simulink model "part1"  (R2024b)
settings: Solver=VariableStepAuto  StartTime=0.0  StopTime=1500  RelTol=1e-3
values from neighbouring files (symbols this model uses):
  A_f = diag([1/t1 1/t2 1/t3])    [reference_model.m]
  Gamma = diag([w1^2, w2^2, w3^2])    [reference_model.m]
  Kd = diag([Kd_t(1,1), Kd_t(2,2), Kd_t(3,3)])    [PID.m]
  Ki = diag([Ki_t(1,1), Ki_t(2,2), Ki_t(3,3)])    [PID.m]
  Kp = diag([Kp_t(1,1), Kp_t(2,2), Kp_t(3,3)])    [PID.m]
  Omega = diag([2*zeta1*w1, 2*zeta2*w2, 2*zeta3*w3])    [reference_model.m]
  step1 = 50    [reference_model.m]
  step2 = 1.4    [reference_model.m]
  step3 = 1.2    [reference_model.m]
  W = diag([10, 1, 1, 10, 1, 1, 1, 1])    [thrust_allocation.m]
  xpos = [thrusters.xposition]    [thrust_allocation.m]
  ypos = [thrusters.yposition]    [thrust_allocation.m]
undefined symbols (not defined in the file or in its folder): alpha, C_pitch, C_roll, C_yaw, Cx, Cy, Cz, Hoerner, magnitude, thrusters, vessel
libraries: simulink x4, marine_gnc x3, marine_hydro x1
settings Model: Creator=jonbjor  LastModifiedBy=audun
settings SolverCC: AlgebraicLoopSolver=TrustRegion
settings DataIOCC: ReturnWorkspaceOutputs=off
settings DebuggingCC: UnconnectedInputMsg=warning  UnconnectedOutputMsg=warning  UnconnectedLineMsg=warning  ArithmeticOperatorsInVariantConditions=warning
settings ModelReferenceCC: EnableRefExpFcnMdlSchedulingChecks=on
settings SFSimCC: SimUseLocalCustomCode=off  CustomCodeUndefinedFunction=UseInterfaceOnly
settings RTWCC: RTWUseLocalCustomCode=off  GPUComputeCapability=3.5  DLArmComputeVersion=19.05

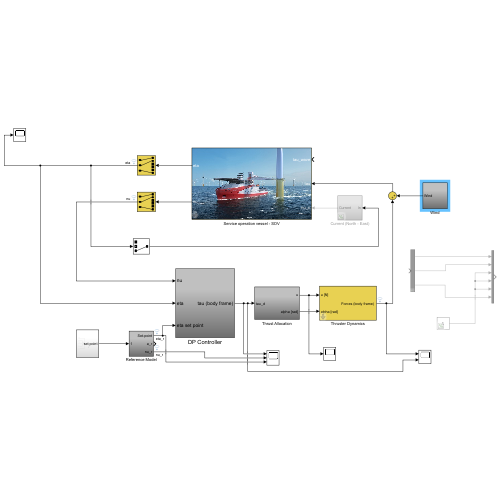
[thumbnail: Simulink's stored preview of the top-level diagram]
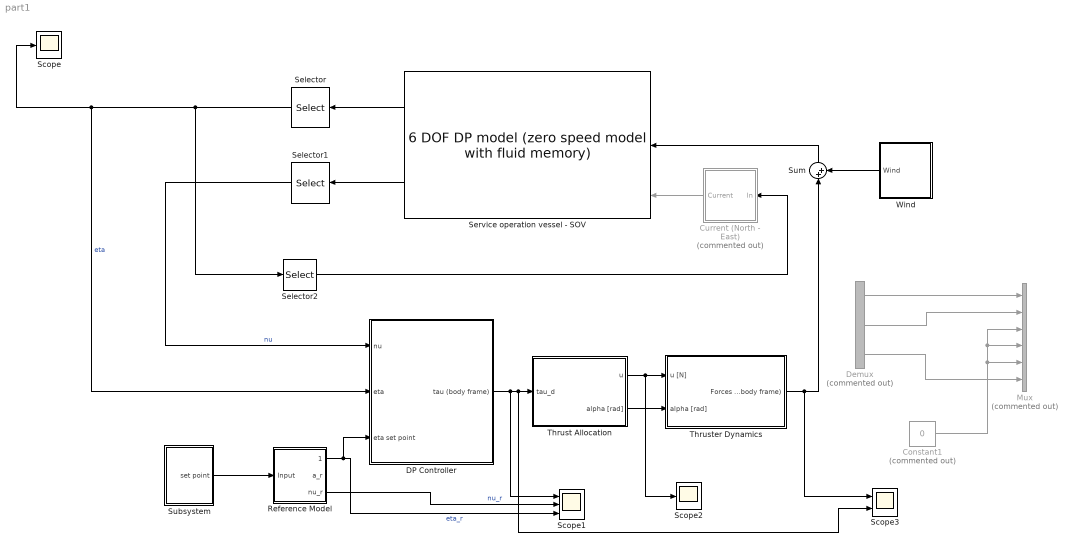
== system part1 ==
  Constant1 : Constant  Commented=on  Value=0
  Current (North - East) : Subsystem  Commented=on
  DP Controller : Subsystem
  Demux : Demux  Commented=on  Outputs=3
  Mux : Mux  Commented=on  Inputs=6
  Reference Model : Subsystem
  Scope : Scope
  Scope1 : Scope  NumInputPorts=3
  Scope2 : Scope
  Scope3 : Scope  NumInputPorts=2
  Selector : Selector  InputPortWidth=6  IndexOptions=Index vector (dialog)  Indices=[1 2 6]  OutputSizes=1
  Selector1 : Selector  InputPortWidth=6  IndexOptions=Index vector (dialog)  Indices=[1 2 6]  OutputSizes=1
  Selector2 : Selector  InputPortWidth=3  IndexOptions=Index vector (dialog)  Indices=[3]  OutputSizes=1
  Service operation vessel - SOV : marine_hydro/Hydro Library/6 DOF DP model  (zero speed model with fluid memory)  ABC=vesselABC  rho=1025  Axc=0.9*vessel.main.T*vessel.main.B  Ayc=0.9*vessel.main.T*vessel.main.Lpp  CX=1  CY_2D=Hoerner(vessel.main.B,vessel.main.T)  Bv=vessel.Bv  mask(6 DOF zero speed model){}
      link override "Integrator1 ": InitialCondition=nu0
      link override Integrator2: InitialCondition=eta0
      settings: SourceProductName=MSS Hydro
      mask Display:
      | image('SOV.jpg');
      | color('white'); port_label('output', 1, 'eta')
      | color('white'); port_label('output', 2, 'nu')
      | color('white'); port_label('input', 1, 'tau_wave')
      | color('white'); port_label('input', 2, 'tau')
      | color('white'); port_label('input', 3, 'nu_c')
  Subsystem : Subsystem
  Sum : Sum  Inputs=|++
  Thrust Allocation : Subsystem
  Thruster Dynamics : Subsystem  mask{thrusterfault=off}
      mask prompts: thrusterfault "Fault on thruster #2 and #4?"
  Wind : Subsystem
  wires:
  Thruster Dynamics/1("Forces (body frame) ") -> Scope3/1, Sum/1
  Service operation vessel - SOV/1 -> Selector/1
  Service operation vessel - SOV/2 -> Selector1/1
  Selector/1 -> Selector2/1, DP Controller/2(eta), Scope/1  "eta"
  Selector1/1 -> DP Controller/1(nu)  "nu"
  DP Controller/1(tau (body frame)) -> Scope1/1, Scope3/2, Thrust Allocation/1(tau_d)
  Wind/1(Wind) -> Sum/2
  Demux/1 -> Mux/1
  Demux/2 -> Mux/2
  Constant1/1 -> Mux/5, Mux/4, Mux/3
  Demux/3 -> Mux/6
  Thrust Allocation/1(u) -> Scope2/1, Thruster Dynamics/1(u [N])
  Thrust Allocation/2(alpha [rad]) -> Thruster Dynamics/2(alpha [rad])
  Sum/1 -> Service operation vessel - SOV/2
  Subsystem/1(set point) -> Reference Model/1(Input)
  Selector2/1 -> Current (North - East)/1(In)
  Current (North - East)/1(Current) -> Service operation vessel - SOV/3
  Reference Model/1(Set-point) -> DP Controller/3(eta set point), Scope1/3  "eta_r"
  Reference Model/3(nu_r) -> Scope1/2  "nu_r"

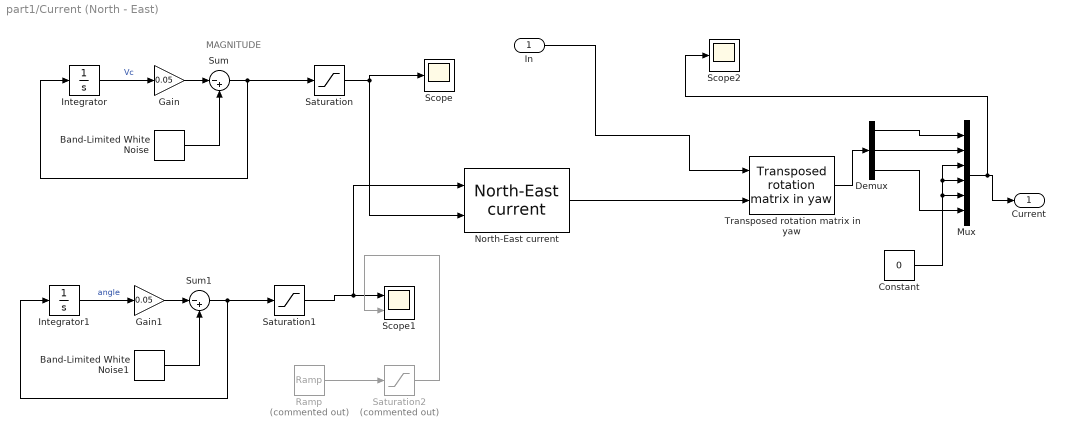
== system part1/Current (North - East) ==
  note: MAGNITUDE
  In : Inport
  Band-Limited White Noise : simulink/Sources/Band-Limited White Noise  Cov=[0.1]  Ts=0.1  seed=[23341]
  Band-Limited White Noise1 : simulink/Sources/Band-Limited White Noise  Cov=[0.1]  Ts=0.1  seed=[23341]
  Constant : Constant  Value=0
  Demux : Demux  Outputs=3
  Gain : Gain  Gain=0.05
  Gain1 : Gain  Gain=0.05
  Integrator : Integrator
  Integrator1 : Integrator
  Mux : Mux  Inputs=6
  North-East current : marine_gnc/Environment/Current/North-East current  SystemSampleTime=-1  VariantActivationTime=update diagram  AllowFlexibleInterface=on  Latency=0  AutoFrameSizeCalculation=off
      settings: SourceProductName=MSS GNC
  Ramp : simulink/Sources/Ramp  Commented=on  slope=0.3  start=0  InitialOutput=180
  Saturation : Saturate  LowerLimit=0.5
  Saturation1 : Saturate  UpperLimit=270  LowerLimit=270
  Saturation2 : Saturate  Commented=on  UpperLimit=270  LowerLimit=0
  Scope : Scope
  Scope1 : Scope  NumInputPorts=2
  Scope2 : Scope
  Sum : Sum  Inputs=|-+
  Sum1 : Sum  Inputs=|-+
  Transposed rotation matrix in yaw : marine_gnc/Models/ Kinematics/Transposed rotation  matrix in yaw
      settings: SourceProductName=MSS GNC
  Current : Outport  VectorParamsAs1DForOutWhenUnconnected=off
  wires:
  Transposed rotation matrix in yaw/1 -> Demux/1
  In/1 -> Transposed rotation matrix in yaw/1
  Demux/1 -> Mux/1
  Band-Limited White Noise1/1 -> Sum1/2
  Integrator/1 -> Gain/1  "Vc"
  Sum/1 -> Saturation/1, Integrator/1
  Gain/1 -> Sum/1
  Integrator1/1 -> Gain1/1  "angle"
  Gain1/1 -> Sum1/1
  Constant/1 -> Mux/5, Mux/4, Mux/3
  Demux/3 -> Mux/6
  Saturation/1 -> Scope/1, North-East current/2
  Saturation1/1 -> North-East current/1, Scope1/1
  Sum1/1 -> Saturation1/1, Integrator1/1
  North-East current/1 -> Transposed rotation matrix in yaw/2
  Band-Limited White Noise/1 -> Sum/2
  Mux/1 -> Scope2/1, Current/1
  Demux/2 -> Mux/2
  Ramp/1 -> Saturation2/1
  Saturation2/1 -> Scope1/2

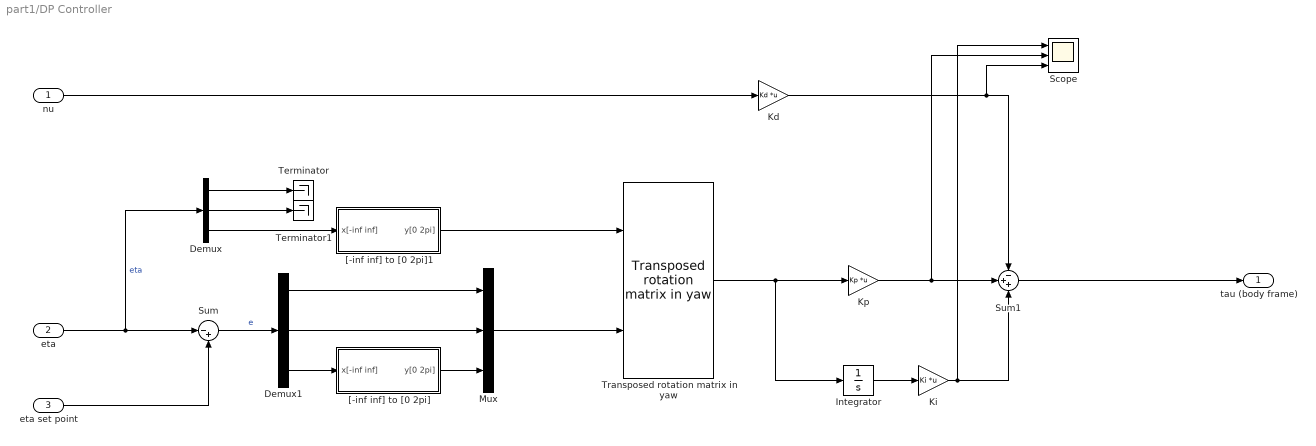
== system part1/DP Controller ==
  nu : Inport
  eta : Inport  Port=2
  eta set point : Inport  Port=3
  Demux : Demux  Outputs=3
  Demux1 : Demux  Outputs=3
  Integrator : Integrator
  Kd : Gain  Gain=Kd  Multiplication=Matrix(K*u)
  Ki : Gain  Gain=Ki  Multiplication=Matrix(K*u)
  Kp : Gain  Gain=Kp  Multiplication=Matrix(K*u)
  Mux : Mux  Inputs=3
  Scope : Scope  NumInputPorts=3
  Sum : Sum  Inputs=|-+
  Sum1 : Sum  Inputs=-++
  Terminator : Terminator
  Terminator1 : Terminator
  Transposed rotation matrix in yaw : marine_gnc/Models/ Kinematics/Transposed rotation  matrix in yaw
      settings: SourceProductName=MSS GNC
  "[-inf inf] to [0 2pi]" : Subsystem
  "[-inf inf] to [0 2pi]1" : Subsystem
  tau (body frame) : Outport  VectorParamsAs1DForOutWhenUnconnected=off
  wires:
  eta set point/1 -> Sum/2
  eta/1 -> Demux/1, Sum/1  "eta"
  Sum/1 -> Demux1/1  "e"
  Demux/1 -> Terminator/1
  Demux/2 -> Terminator1/1
  Demux/3 -> "[-inf inf] to [0 2pi]1"/1(x[-inf inf])
  Demux1/2 -> Mux/2
  Demux1/3 -> "[-inf inf] to [0 2pi]"/1(x[-inf inf])
  Demux1/1 -> Mux/1
  "[-inf inf] to [0 2pi]"/1(y[0 2pi]) -> Mux/3
  Integrator/1 -> Ki/1
  Ki/1 -> Scope/1, Sum1/3
  Kp/1 -> Scope/2, Sum1/2
  Kd/1 -> Scope/3, Sum1/1
  Sum1/1 -> tau (body frame)/1
  Mux/1 -> Transposed rotation matrix in yaw/2
  Transposed rotation matrix in yaw/1 -> Integrator/1, Kp/1
  nu/1 -> Kd/1
  "[-inf inf] to [0 2pi]1"/1(y[0 2pi]) -> Transposed rotation matrix in yaw/1

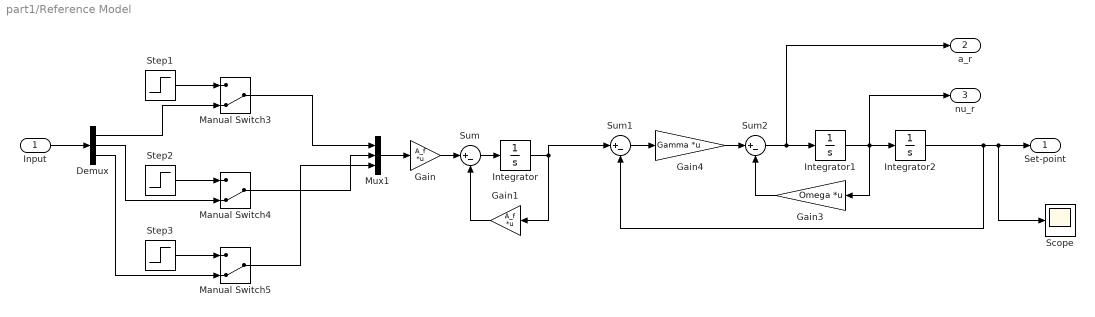
== system part1/Reference Model ==
  Input : Inport
  Demux : Demux  Outputs=3
  Gain : Gain  Gain=A_f  Multiplication=Matrix(K*u)
  Gain1 : Gain  Gain=A_f  Multiplication=Matrix(K*u)
  Gain3 : Gain  Gain=Omega  Multiplication=Matrix(K*u)
  Gain4 : Gain  Gain=Gamma  Multiplication=Matrix(K*u)
  Integrator : Integrator
  Integrator1 : Integrator
  Integrator2 : Integrator
  Manual Switch3 : ManualSwitch  CurrentSetting=0
  Manual Switch4 : ManualSwitch  CurrentSetting=0
  Manual Switch5 : ManualSwitch  CurrentSetting=0
  Mux1 : Mux  Inputs=3
  Scope : Scope
  Step1 : Step  After=step1  SampleTime=1
  Step2 : Step  After=step2  SampleTime=1
  Step3 : Step  After=step3  SampleTime=1
  Sum : Sum  Inputs=|+-
  Sum1 : Sum  Inputs=|+-
  Sum2 : Sum  Inputs=|+-
  Set-point : Outport  VectorParamsAs1DForOutWhenUnconnected=off
  a_r : Outport  Port=2
  nu_r : Outport  Port=3
  wires:
  Manual Switch3/1 -> Mux1/1
  Demux/1 -> Manual Switch3/2
  Mux1/1 -> Gain/1
  Gain4/1 -> Sum2/1
  Integrator/1 -> Sum1/1, Gain1/1
  Gain/1 -> Sum/1
  Step2/1 -> Manual Switch4/1
  Sum/1 -> Integrator/1
  Integrator2/1 -> Sum1/2, Scope/1, Set-point/1
  Gain3/1 -> Sum2/2
  Gain1/1 -> Sum/2
  Demux/3 -> Manual Switch5/2
  Manual Switch5/1 -> Mux1/3
  Demux/2 -> Manual Switch4/2
  Manual Switch4/1 -> Mux1/2
  Input/1 -> Demux/1
  Step1/1 -> Manual Switch3/1
  Step3/1 -> Manual Switch5/1
  Integrator1/1 -> Gain3/1, nu_r/1, Integrator2/1
  Sum2/1 -> a_r/1, Integrator1/1
  Sum1/1 -> Gain4/1

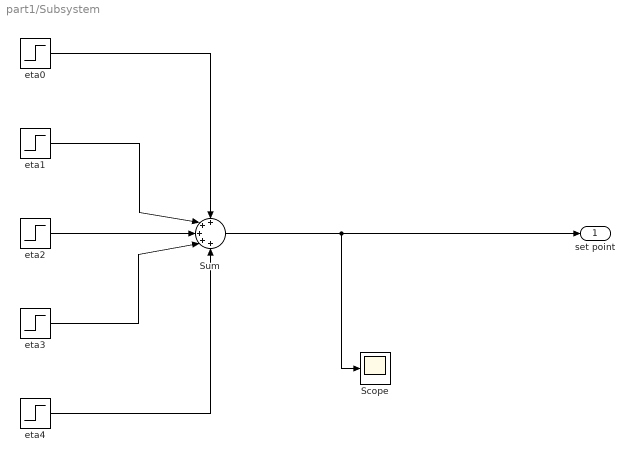
== system part1/Subsystem ==
  Scope : Scope
  Sum : Sum  Inputs=+++++
  eta0 : Step  Before=[0, 0 , 0]  After=[50, 0, 0]  SampleTime=0
  eta1 : Step  Time=301  Before=[0, 0 , 0]  After=[0, -50, 0]  SampleTime=0
  eta2 : Step  Time=601  Before=[0, 0, 0]  After=[0, 0, -pi/4]  SampleTime=0
  eta3 : Step  Time=901  Before=[0, 0, 0]  After=[-50, 0, 0]  SampleTime=0
  eta4 : Step  Time=1201  Before=[0, 0, 0]  After=[0, 50, pi/4]  SampleTime=0
  set point : Outport
  wires:
  Sum/1 -> Scope/1, set point/1
  eta0/1 -> Sum/1
  eta1/1 -> Sum/2
  eta2/1 -> Sum/3
  eta3/1 -> Sum/4
  eta4/1 -> Sum/5

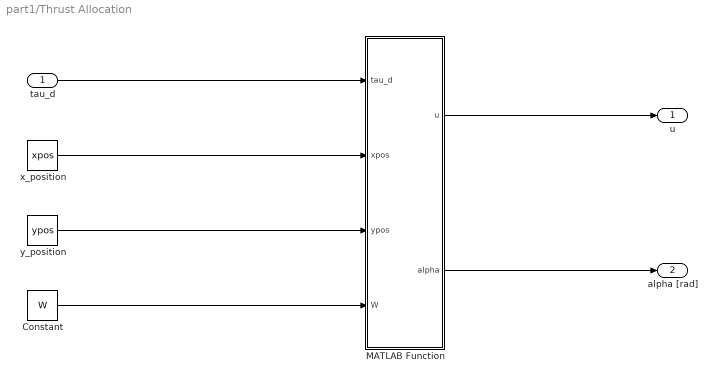
== system part1/Thrust Allocation ==
  tau_d : Inport
  Constant : Constant  Value=W
  MATLAB Function : MATLAB Function  TreatAsAtomicUnit=on
  x_position : Constant  Value=xpos
  y_position : Constant  Value=ypos
  u : Outport  VectorParamsAs1DForOutWhenUnconnected=off
  alpha [rad] : Outport  Port=2  VectorParamsAs1DForOutWhenUnconnected=off
  wires:
  tau_d/1 -> MATLAB Function/1(tau_d)
  x_position/1 -> MATLAB Function/2(xpos)
  y_position/1 -> MATLAB Function/3(ypos)
  MATLAB Function/2(alpha) -> alpha [rad]/1
  MATLAB Function/1(u) -> u/1
  Constant/1 -> MATLAB Function/4(W)

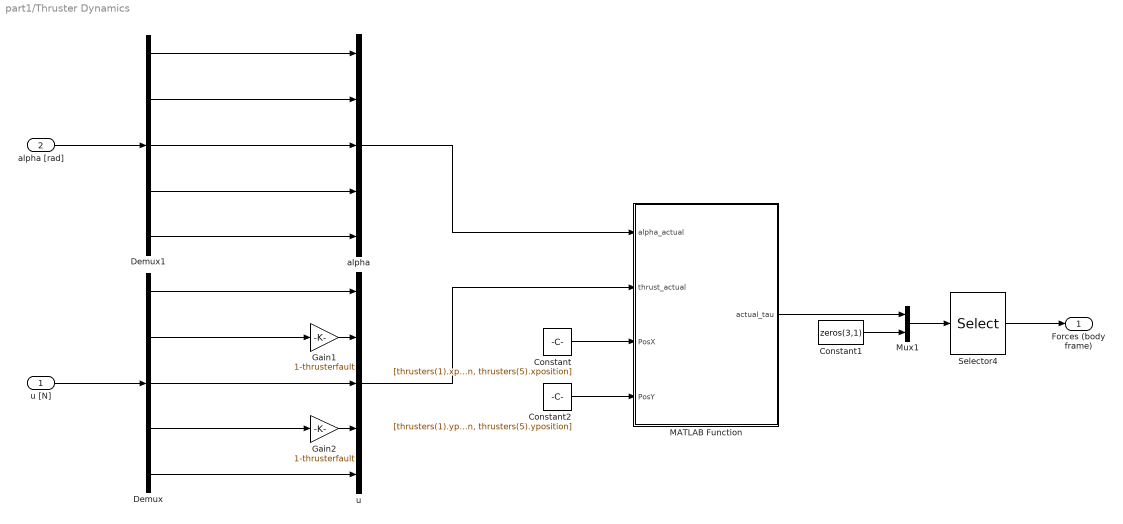
== system part1/Thruster Dynamics ==
  u [N] : Inport
  alpha [rad] : Inport  Port=2
  Constant : Constant  Value=[thrusters(1).xposition, thrusters(2).xposition, thrusters(3).xposition, thrusters(4).xposition, thrusters(5).xposition]
  Constant1 : Constant  Value=zeros(3,1)
  Constant2 : Constant  Value=[thrusters(1).yposition, thrusters(2).yposition, thrusters(3).yposition, thrusters(4).yposition, thrusters(5).yposition]
  Demux : Demux  Outputs=5
  Demux1 : Demux  Outputs=5
  Gain1 : Gain  Gain=1-thrusterfault
  Gain2 : Gain  Gain=1-thrusterfault
  MATLAB Function : MATLAB Function  TreatAsAtomicUnit=on
  Mux1 : Mux  Inputs=2
  Selector4 : Selector  InputPortWidth=6  IndexOptions=Index vector (dialog)  Indices=[1 2 4 5 6 3]  OutputSizes=1
  alpha : Mux  Inputs=5
  u : Mux  Inputs=5
  "Forces (body frame) " : Outport  VectorParamsAs1DForOutWhenUnconnected=off
  wires:
  Mux1/1 -> Selector4/1
  Constant1/1 -> Mux1/2
  Selector4/1 -> "Forces (body frame) "/1
  Gain1/1 -> u/2
  u [N]/1 -> Demux/1
  alpha [rad]/1 -> Demux1/1
  Constant/1 -> MATLAB Function/3(PosX)
  Constant2/1 -> MATLAB Function/4(PosY)
  u/1 -> MATLAB Function/2(thrust_actual)
  alpha/1 -> MATLAB Function/1(alpha_actual)
  MATLAB Function/1(actual_tau) -> Mux1/1
  Demux1/1 -> alpha/1
  Gain2/1 -> u/4
  Demux/1 -> u/1
  Demux/2 -> Gain1/1
  Demux/3 -> u/3
  Demux/4 -> Gain2/1
  Demux/5 -> u/5
  Demux1/2 -> alpha/2
  Demux1/4 -> alpha/4
  Demux1/5 -> alpha/5
  Demux1/3 -> alpha/3

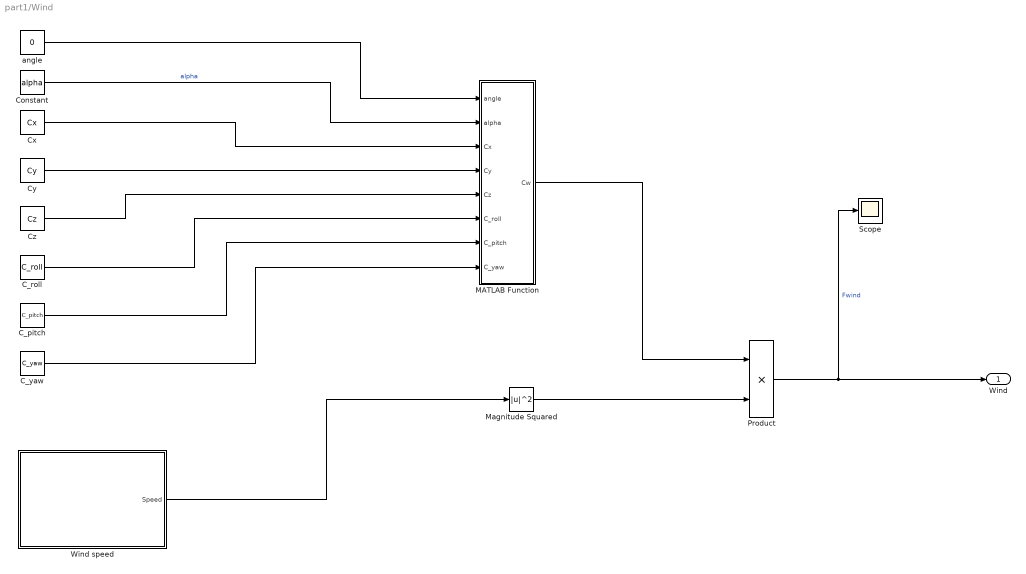
== system part1/Wind ==
  C_pitch : Constant  Value=C_pitch
  C_roll : Constant  Value=C_roll
  C_yaw : Constant  Value=C_yaw
  Constant : Constant  Value=alpha
  Cx : Constant  Value=Cx
  Cy : Constant  Value=Cy
  Cz : Constant  Value=Cz
  MATLAB Function : MATLAB Function  TreatAsAtomicUnit=on
  Magnitude Squared : Math  Operator=magnitude^2
  Product : Product
  Scope : Scope
  Wind speed : Subsystem
  angle : Constant  Value=0
  Wind : Outport  VectorParamsAs1DForOutWhenUnconnected=off
  wires:
  Cz/1 -> MATLAB Function/5(Cz)
  Cy/1 -> MATLAB Function/4(Cy)
  Cx/1 -> MATLAB Function/3(Cx)
  C_yaw/1 -> MATLAB Function/8(C_yaw)
  C_roll/1 -> MATLAB Function/6(C_roll)
  C_pitch/1 -> MATLAB Function/7(C_pitch)
  Magnitude Squared/1 -> Product/2
  Product/1 -> Wind/1, Scope/1  "Fwind"
  MATLAB Function/1(Cw) -> Product/1
  Constant/1 -> MATLAB Function/2(alpha)  "alpha"
  Wind speed/1(Speed) -> Magnitude Squared/1
  angle/1 -> MATLAB Function/1(angle)

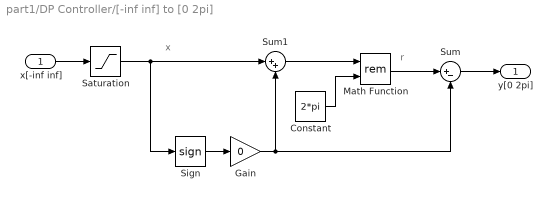
== system part1/DP Controller/[-inf inf] to [0 2pi] ==
  note: r
  note: x
  x[-inf inf] : Inport
  Constant : Constant  Value=2*pi
  Gain : Gain  Gain=0  SaturateOnIntegerOverflow=on  OutDataTypeStr=Inherit: Same as input  ParamDataTypeStr=Inherit: Same as input
  Math Function : Math  Operator=rem  SignedPower=on
  Saturation : Saturate  UpperLimit=1e10  LowerLimit=-1e10
  Sign : Signum
  Sum : Sum  Inputs=|+-  SaturateOnIntegerOverflow=on
  Sum1 : Sum  Inputs=|++  SaturateOnIntegerOverflow=on
  y[0 2pi] : Outport
  wires:
  Saturation/1 -> Sum1/1, Sign/1
  Constant/1 -> Math Function/2
  x[-inf inf]/1 -> Saturation/1
  Math Function/1 -> Sum/1
  Sum/1 -> y[0 2pi]/1
  Gain/1 -> Sum/2, Sum1/2
  Sign/1 -> Gain/1
  Sum1/1 -> Math Function/1

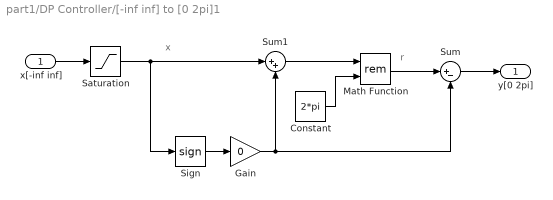
== system part1/DP Controller/[-inf inf] to [0 2pi]1 ==
  note: r
  note: x
  x[-inf inf] : Inport
  Constant : Constant  Value=2*pi
  Gain : Gain  Gain=0  SaturateOnIntegerOverflow=on  OutDataTypeStr=Inherit: Same as input  ParamDataTypeStr=Inherit: Same as input
  Math Function : Math  Operator=rem  SignedPower=on
  Saturation : Saturate  UpperLimit=1e10  LowerLimit=-1e10
  Sign : Signum
  Sum : Sum  Inputs=|+-  SaturateOnIntegerOverflow=on
  Sum1 : Sum  Inputs=|++  SaturateOnIntegerOverflow=on
  y[0 2pi] : Outport
  wires:
  Saturation/1 -> Sum1/1, Sign/1
  Constant/1 -> Math Function/2
  x[-inf inf]/1 -> Saturation/1
  Math Function/1 -> Sum/1
  Sum/1 -> y[0 2pi]/1
  Gain/1 -> Sum/2, Sum1/2
  Sign/1 -> Gain/1
  Sum1/1 -> Math Function/1

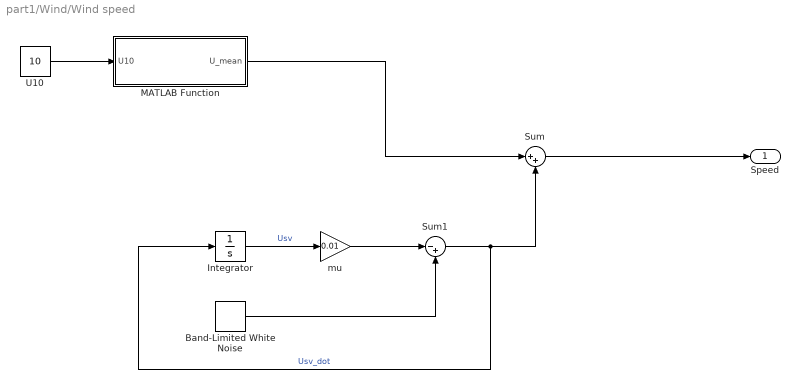
== system part1/Wind/Wind speed ==
  Band-Limited White Noise : simulink/Sources/Band-Limited White Noise  Cov=[0.1]  Ts=0.1  seed=[23341]
  Integrator : Integrator
  MATLAB Function : MATLAB Function  TreatAsAtomicUnit=on
  Sum : Sum  Inputs=|++
  Sum1 : Sum  Inputs=|-+
  U10 : Constant  Value=10
  mu : Gain  Gain=0.01
  Speed : Outport
  wires:
  U10/1 -> MATLAB Function/1(U10)
  Sum/1 -> Speed/1
  mu/1 -> Sum1/1
  Integrator/1 -> mu/1  "Usv"
  Band-Limited White Noise/1 -> Sum1/2
  Sum1/1 -> Integrator/1, Sum/2  "Usv_dot"
  MATLAB Function/1(U_mean) -> Sum/1

== matlab function part1/Thrust Allocation/MATLAB Function ==
  data: tau_d input; u output; xpos input; ypos input; alpha output; W input
function [u,alpha] = fcn(tau_d, xpos, ypos, W)

l_1 = xpos(1);
l_2x = xpos(2);
l_2y = ypos(2);
l_3 = xpos(3);
l_4x = xpos(4);
l_4y = ypos(4);
l_5x = xpos(5);
l_5y = ypos(5);

B = [[0, 0, 1, 0, 1, 0, 1, 0];
    [1, 1, 0, 1, 0, 1, 0, 1];
    [l_1, l_2y, l_2x, l_3, l_4y, l_4x, l_5y, l_5x]];

W_inv = inv(W);
B_pseudo = pinv(B);
C = W_inv * B_pseudo * inv(B*W_inv*B_pseudo);

u_temp = C*tau_d;

a1 = pi/2;
a2 = atan2(u_temp(3), u_temp(2));
a3 = pi/2;
a4 = atan2(u_temp(6), u_temp(5));
a5 = atan2(u_temp(8), u_temp(7));

alpha = [a1; a2; a3; a4; a5];

u = [u_temp(1), sqrt(u_temp(2)^2 + u_temp(3)^2), u_temp(4), sqrt(u_temp(5)^2 + u_temp(6)^2), sqrt(u_temp(7)^2 + u_temp(8)^2)];


end

== matlab function part1/Wind/MATLAB Function ==
  data: Cw output; angle input; alpha input; Cx input; Cy input; Cz input; C_roll input; C_pitch input; C_yaw input
function Cw = fcn(angle, alpha, Cx, Cy, Cz, C_roll, C_pitch, C_yaw)

Cw = zeros(6, 1);

index = find(abs(alpha - angle) == 0);

Cw(1) = Cx(index);
Cw(2) = Cy(index);
Cw(3) = Cz(index);
Cw(4) = C_roll(index);
Cw(5) = C_pitch(index);
Cw(6) = C_yaw(index);
end

== matlab function part1/Wind/Wind speed/MATLAB Function ==
  data: U10 input; U_mean output
function U_mean = fcn(U10)

K = 0.003;
z = 3;
z0 = 10*exp(-2/(5*sqrt(K)));

U_mean = U10*(5/2)*sqrt(K)*log(z/z0);

end

== matlab function part1/Thruster Dynamics/MATLAB Function ==
  data: alpha_actual input; thrust_actual input; actual_tau output; PosX input; PosY input
function actual_tau   = fcn(alpha_actual,thrust_actual,PosX,PosY)

    Alpha_surge =[cos(alpha_actual(1)) cos(alpha_actual(2)) cos(alpha_actual(3)) cos(alpha_actual(4)) cos(alpha_actual(5))];  
    Alpha_sway = [sin(alpha_actual(1)) sin(alpha_actual(2)) sin(alpha_actual(3)) sin(alpha_actual(4)) sin(alpha_actual(5))];
    Alpha_yaw = [sin(alpha_actual(1))*PosX(1)-cos(alpha_actual(1))*PosY(1) sin(alpha_actual(2))*PosX(2)-cos(alpha_actual(2))*PosY(2) ...
                 sin(alpha_actual(3))*PosX(3)-cos(alpha_actual(3))*PosY(3) sin(alpha_actual(4))*PosX(4)-cos(alpha_actual(4))*PosY(4) ...
                 sin(alpha_actual(5))*PosX(5)-cos(alpha_actual(5))*PosY(5)];

    actual_tau = [Alpha_surge; Alpha_sway; Alpha_yaw]*thrust_actual;
end
